simulink model "RenanArdaCarlak_ShakeWeightDumbbell"  (R2019b)
settings: Solver=VariableStepAuto  StartTime=0.0  StopTime=40  RelTol=1e-3
libraries: vrlib x4
settings Model: EnablePacing=on  PacingRate=0.900000  Creator=ARDA  LastModifiedBy=ARDA

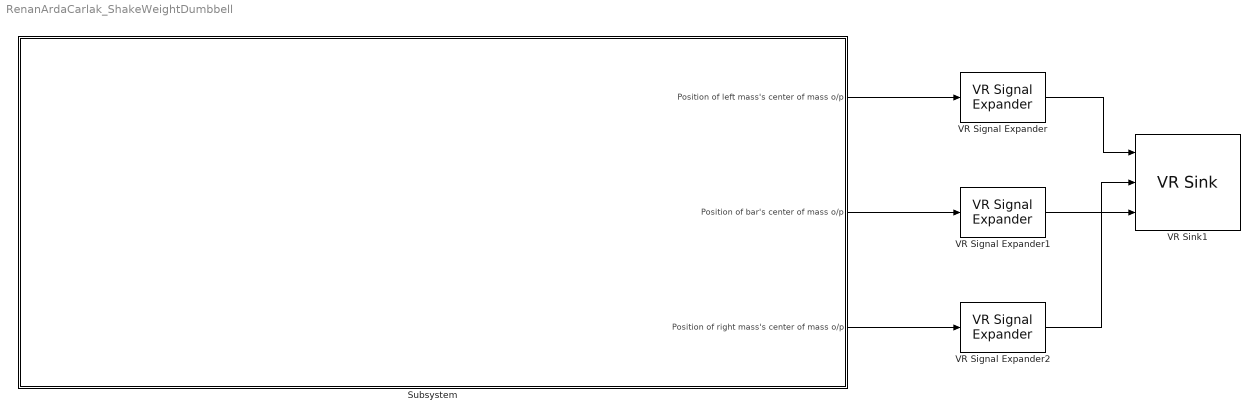
== system RenanArdaCarlak_ShakeWeightDumbbell ==
  Subsystem : Subsystem  mask{amplitude=-0.001, frequency=0.32, m2=0.5, BarThickness=0.05, m1=1, LeftThickness=0.03, LeftLength=0.1, LeftSpringConstant=1, m3=1, RightThickness=0.03, RightLength=0.1, RightSpringConstant=1}
      mask DialogControl DescGroupVar Prompt: Shake Weight Dumble
      mask DialogControl DescTextVar Prompt: You can set all parameters in here.
      mask DialogControl Control2 Prompt: Amplitude of Applied Force [N]
      mask DialogControl Control3 Prompt: Frequency of Applied Force (in Hertz)
      mask DialogControl Control5 Prompt: Weight of Dumbble Bar [kg]
      mask DialogControl Control16 Prompt: Thickness of Bar [m]
      mask DialogControl Control4 Prompt: Left Side Weigth of Dumbble [kg]
      mask DialogControl Control12 Prompt: Thickness of Left Side Weight [m]
      mask DialogControl Control6 Prompt: Length between the middle of the Dumbble Bar and Left Weight of Dumbble [m]
      mask DialogControl Control8 Prompt: Spring Constant of Left Spring [kg/s^2]
      mask DialogControl Control10 Prompt: Right Side Weight of Dumbble [kg]
      mask DialogControl Control13 Prompt: Thickness of Right Side Weight [m]
      mask DialogControl Control7 Prompt: Length between the middle of the Dumbble Bar and Right Weight of Dumbble [m]
      mask DialogControl Control9 Prompt: Spring Constant of Right Spring [kg/s^2]
  VR Signal Expander : vrlib/VR Signal Expander  outwidth=3  outidx=[1]
      settings: SourceProductName=Simulink
  VR Signal Expander1 : vrlib/VR Signal Expander  outwidth=3  outidx=[1]
      settings: SourceProductName=Simulink
  VR Signal Expander2 : vrlib/VR Signal Expander  outwidth=3  outidx=[1]
      settings: SourceProductName=Simulink
  VR Sink1 : vrlib/VR Sink  InstantiateOnLoad=on  SampleTime=0.1  ViewEnable=on  RemoteChange=off  RemoteView=off  FieldsWritten=LeftWeight.translation.3.1.1.double#RightWeight.translation.3.1.1.double#Bar.translation.3.1.1.double  WorldFileName=RenanArdaCarlak_ShakeWeightDumbbell.WRL  AutoView=off  VideoDimensions=[]  AllowVariableSize=off
      settings: SourceProductName=Simulink
  wires:
  Subsystem/1(Position of left mass's center of mass o/p) -> VR Signal Expander/1
  Subsystem/2(Position of bar's center of mass o/p) -> VR Signal Expander1/1
  Subsystem/3(Position of right mass's center of mass o/p) -> VR Signal Expander2/1
  VR Signal Expander1/1 -> VR Sink1/3
  VR Signal Expander/1 -> VR Sink1/1
  VR Signal Expander2/1 -> VR Sink1/2

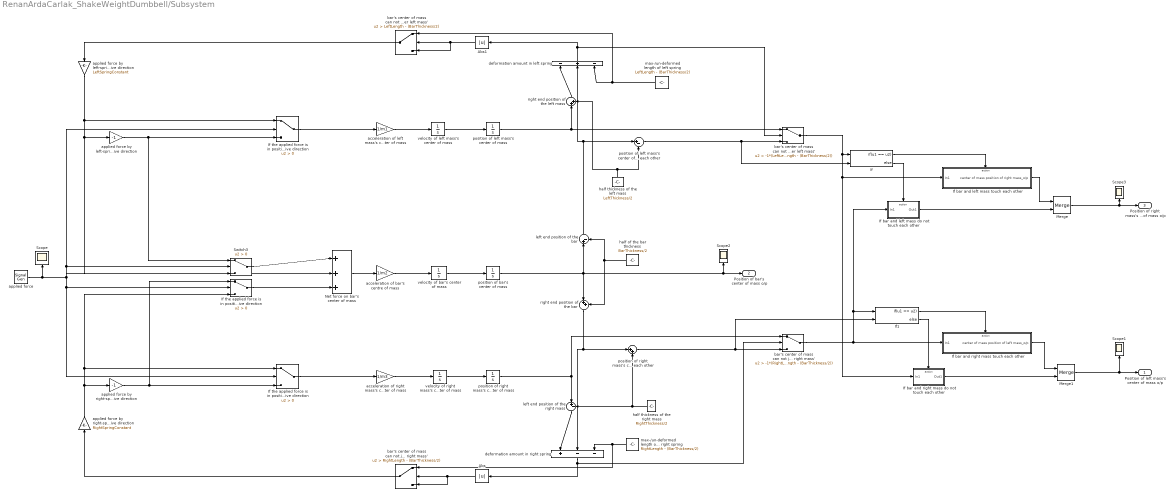
== system RenanArdaCarlak_ShakeWeightDumbbell/Subsystem ==
  "   left end position of the bar" : Sum  Inputs=|+-
  "  left end position of the right mass" : Sum  Inputs=|+-
  "  right end position of the left mass" : Sum  Inputs=|++
  Abs : Abs
  Abs1 : Abs
  If : If  NumInputs=2  IfExpression=u1 == u2
  If bar and left mass do not touch each other : Subsystem  TreatAsAtomicUnit=on
  If bar and left mass touch each other : Subsystem  TreatAsAtomicUnit=on
  If bar and right mass do not touch each other : Subsystem  TreatAsAtomicUnit=on
  If bar and right mass touch each other : Subsystem  TreatAsAtomicUnit=on
  "If the applied force is in positive direction, then, the left and right springs apply forces to the bar's center of mass in negative direction" : Switch  Criteria=u2 > Threshold
  "If the applied force is in positive direction, then, the left-spring applies force to the left mass in positive direction" : Switch  Criteria=u2 > Threshold
  "If the applied force is in positive direction, then, the right-spring applies force to the right mass in positive direction" : Switch  Criteria=u2 > Threshold
  If1 : If  NumInputs=2  IfExpression=u1 == u2
  Merge : Merge
  Merge1 : Merge
  Net force on bar's center of mass : Sum  Inputs=|+++
  Scope{,1..3} (4 alike) : Scope
  Switch3 : Switch  Criteria=u2 > Threshold
  "acceleration of bar's centre of mass  " : Gain  Gain=1/m2
  acceleration of left mass's center of mass : Gain  Gain=1/m1
  acceleration of right mass's center of mass : Gain  Gain=1/m3
  applied force : SignalGenerator  WaveForm=square  Amplitude=amplitude  Frequency=frequency
  applied force by left-spring in negative direction : Gain  Gain=-1
  applied force by left-spring in positive direction : Gain  Gain=LeftSpringConstant
  applied force by right-spring in negative direction : Gain  Gain=-1
  applied force by right-spring in positive direction : Gain  Gain=RightSpringConstant
  bar's center of mass can not jump over left mass' : Switch  Criteria=u2 > Threshold  Threshold=-1*(LeftLength - (BarThickness/2))
  "bar's center of mass can not jump over left mass'  " : Switch  Criteria=u2 > Threshold  Threshold=LeftLength - (BarThickness/2)
  bar's center of mass can not jump over right mass' : Switch  Criteria=u2 > Threshold  Threshold=RightLength - (BarThickness/2)
  "bar's center of mass can not jump over right mass'  " : Switch  Criteria=u2 > Threshold  Threshold=-1*(RightLength - (BarThickness/2))
  deformation amount in left spring : Sum  Inputs=|-+-
  deformation amount in right spring : Sum  Inputs=|+--
  half of the bar thickness : Constant  Value=BarThickness/2
  half thickness of the left mass : Constant  Value=LeftThickness/2
  half thickness of the right mass : Constant  Value=RightThickness/2
  max-/un-deformed length of left spring : Constant  Value=LeftLength - (BarThickness/2)
  max-/un-deformed length of right spring : Constant  Value=RightLength - (BarThickness/2)
  position of bar's center of mass : Integrator
  position of left mass's center of mass : Integrator  InitialCondition=0-LeftLength-(LeftThickness/2)
  "position of left mass's center of mass, in case of bar and left mass touch each other" : Sum  Inputs=|+-
  position of right mass's center of mass : Integrator  InitialCondition=LeftLength+(LeftThickness/2)
  "position of right mass's center of mass, in case of bar and right mass touch each other" : Sum  Inputs=|++
  right end position of the bar : Sum  Inputs=|++
  velocity of bar's center of mass : Integrator
  velocity of left mass's center of mass : Integrator
  velocity of right mass's center of mass : Integrator
  Position of left mass's center of mass o/p : Outport
  Position of bar's center of mass o/p : Outport  Port=2
  Position of right mass's center of mass o/p : Outport  Port=3
  wires:
  applied force by right-spring in positive direction/1 -> applied force by right-spring in negative direction/1, "If the applied force is in positive direction, then, the right-spring applies force to the right mass in positive direction"/1, "If the applied force is in positive direction, then, the left and right springs apply forces to the bar's center of mass in negative direction"/3
  acceleration of right mass's center of mass/1 -> velocity of right mass's center of mass/1
  velocity of left mass's center of mass/1 -> position of left mass's center of mass/1
  "If the applied force is in positive direction, then, the right-spring applies force to the right mass in positive direction"/1 -> acceleration of right mass's center of mass/1
  Net force on bar's center of mass/1 -> "acceleration of bar's centre of mass  "/1
  velocity of right mass's center of mass/1 -> position of right mass's center of mass/1
  velocity of bar's center of mass/1 -> position of bar's center of mass/1
  applied force by left-spring in positive direction/1 -> "If the applied force is in positive direction, then, the left-spring applies force to the left mass in positive direction"/1, applied force by left-spring in negative direction/1, Switch3/3
  "acceleration of bar's centre of mass  "/1 -> velocity of bar's center of mass/1
  "If the applied force is in positive direction, then, the left and right springs apply forces to the bar's center of mass in negative direction"/1 -> Net force on bar's center of mass/3
  applied force/1 -> "If the applied force is in positive direction, then, the right-spring applies force to the right mass in positive direction"/2, "If the applied force is in positive direction, then, the left and right springs apply forces to the bar's center of mass in negative direction"/2, Net force on bar's center of mass/2, Switch3/2, "If the applied force is in positive direction, then, the left-spring applies force to the left mass in positive direction"/2, Scope/1
  applied force by right-spring in negative direction/1 -> "If the applied force is in positive direction, then, the right-spring applies force to the right mass in positive direction"/3, "If the applied force is in positive direction, then, the left and right springs apply forces to the bar's center of mass in negative direction"/1
  acceleration of left mass's center of mass/1 -> velocity of left mass's center of mass/1
  max-/un-deformed length of right spring/1 -> deformation amount in right spring/3, bar's center of mass can not jump over right mass'/1
  deformation amount in left spring/1 -> Abs1/1, bar's center of mass can not jump over left mass'/2
  "If the applied force is in positive direction, then, the left-spring applies force to the left mass in positive direction"/1 -> acceleration of left mass's center of mass/1
  position of left mass's center of mass/1 -> "  right end position of the left mass"/1, bar's center of mass can not jump over left mass'/1
  position of right mass's center of mass/1 -> "bar's center of mass can not jump over right mass'  "/1, "  left end position of the right mass"/1
  applied force by left-spring in negative direction/1 -> "If the applied force is in positive direction, then, the left-spring applies force to the left mass in positive direction"/3, Switch3/1
  deformation amount in right spring/1 -> Abs/1, "bar's center of mass can not jump over right mass'  "/2
  Switch3/1 -> Net force on bar's center of mass/1
  position of bar's center of mass/1 -> right end position of the bar/1, Position of bar's center of mass o/p/1, Scope2/1, "   left end position of the bar"/1
  half thickness of the left mass/1 -> "  right end position of the left mass"/2, "position of left mass's center of mass, in case of bar and left mass touch each other"/2
  "  right end position of the left mass"/1 -> deformation amount in left spring/1
  half thickness of the right mass/1 -> "  left end position of the right mass"/2, "position of right mass's center of mass, in case of bar and right mass touch each other"/2
  "  left end position of the right mass"/1 -> deformation amount in right spring/1
  half of the bar thickness/1 -> right end position of the bar/2, "   left end position of the bar"/2
  "   left end position of the bar"/1 -> deformation amount in left spring/2, "position of left mass's center of mass, in case of bar and left mass touch each other"/1
  right end position of the bar/1 -> deformation amount in right spring/2, "position of right mass's center of mass, in case of bar and right mass touch each other"/1
  Abs/1 -> bar's center of mass can not jump over right mass'/3, bar's center of mass can not jump over right mass'/2
  bar's center of mass can not jump over right mass'/1 -> applied force by right-spring in positive direction/1
  Abs1/1 -> "bar's center of mass can not jump over left mass'  "/3, "bar's center of mass can not jump over left mass'  "/2
  max-/un-deformed length of left spring/1 -> deformation amount in left spring/3, "bar's center of mass can not jump over left mass'  "/1
  "bar's center of mass can not jump over left mass'  "/1 -> applied force by left-spring in positive direction/1
  "position of right mass's center of mass, in case of bar and right mass touch each other"/1 -> If1/2, "bar's center of mass can not jump over right mass'  "/3
  "position of left mass's center of mass, in case of bar and left mass touch each other"/1 -> bar's center of mass can not jump over left mass'/3, If/2
  bar's center of mass can not jump over left mass'/1 -> If bar and left mass touch each other/1(In1), If bar and right mass do not touch each other/1(In1), If/1
  If/1 -> If bar and left mass touch each other/Action
  If/2 -> If bar and left mass do not touch each other/Action
  "bar's center of mass can not jump over right mass'  "/1 -> If bar and right mass touch each other/1(In1), If1/1, If bar and left mass do not touch each other/1(In1)
  If bar and left mass touch each other/1(center of mass position of right mass_o/p) -> Merge/1
  If bar and left mass do not touch each other/1(Out1) -> Merge/2
  Merge/1 -> Scope3/1, Position of right mass's center of mass o/p/1
  If1/1 -> If bar and right mass touch each other/Action
  If1/2 -> If bar and right mass do not touch each other/Action
  If bar and right mass do not touch each other/1(Out1) -> Merge1/2
  If bar and right mass touch each other/1(center of mass position of left mass_o/p) -> Merge1/1
  Merge1/1 -> Position of left mass's center of mass o/p/1, Scope1/1

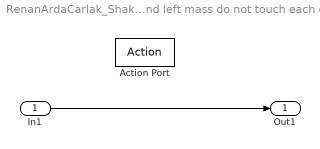
== system RenanArdaCarlak_ShakeWeightDumbbell/Subsystem/If bar and left mass do not touch each other ==
  In1 : Inport
  Action Port : ActionPort  ActionPortLabel=else
  Out1 : Outport
  wires:
  In1/1 -> Out1/1

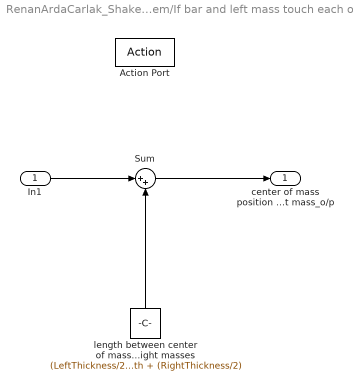
== system RenanArdaCarlak_ShakeWeightDumbbell/Subsystem/If bar and left mass touch each other ==
  In1 : Inport
  Action Port : ActionPort  ActionPortLabel=if(u1 == u2)
  Sum : Sum  Inputs=|++
  "length between center of masses of left and right masses " : Constant  Value=(LeftThickness/2) + LeftLength + RightLength + (RightThickness/2)
  center of mass position of right mass_o/p : Outport
  wires:
  In1/1 -> Sum/1
  Sum/1 -> center of mass position of right mass_o/p/1
  "length between center of masses of left and right masses "/1 -> Sum/2

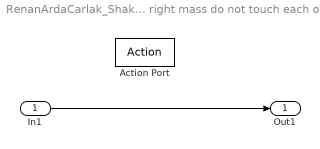
== system RenanArdaCarlak_ShakeWeightDumbbell/Subsystem/If bar and right mass do not touch each other ==
  In1 : Inport
  Action Port : ActionPort  ActionPortLabel=else
  Out1 : Outport
  wires:
  In1/1 -> Out1/1

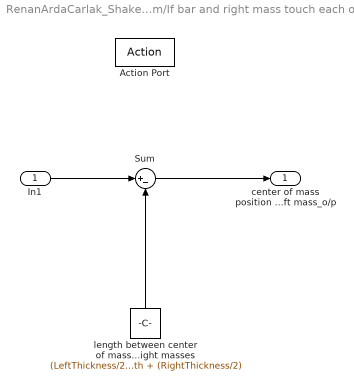
== system RenanArdaCarlak_ShakeWeightDumbbell/Subsystem/If bar and right mass touch each other ==
  In1 : Inport
  Action Port : ActionPort  ActionPortLabel=if(u1 == u2)
  Sum : Sum  Inputs=|+-
  "length between center of masses of left and right masses " : Constant  Value=(LeftThickness/2) + LeftLength + RightLength + (RightThickness/2)
  center of mass position of left mass_o/p : Outport
  wires:
  "length between center of masses of left and right masses "/1 -> Sum/2
  Sum/1 -> center of mass position of left mass_o/p/1
  In1/1 -> Sum/1
